simulink model "TEST_IPM_2_0"  (R2019b)
settings: configuration reference "Configuration" (kept outside this file)
PreLoadFcn:
  | RTWConfigurationCB('preloadfcn', bdroot);
values from neighbouring files (symbols this model uses):
  MParamFbase = 200.0    [TEST_IPM_LIB.sldd]
  MParamIbase = 360.0    [TEST_IPM_LIB.sldd]
  MParamLd = 0.002    [TEST_IPM_LIB.sldd]
  MParamLq = 0.002    [TEST_IPM_LIB.sldd]
  MParamRs = 1.15    [TEST_IPM_LIB.sldd]
  PWM_TPBRD_HALF = 5000.0    [TEST_IPM_LIB.sldd]
  Ts_10kHz = 0.0001    [TEST_IPM_LIB.sldd]
  Ts_1kHz = 0.001    [TEST_IPM_LIB.sldd]
undefined symbols (not defined in the file or in its folder): Down, GPTRIP1SEL, GPTRIP2SEL, TZ1, TZ2, Up
libraries: c280xlib x66, c2837xDlib x18, c2802xlib x10, powerlib_meascontrol x9, dsparch4 x4, c2000lib x1, c2806xlib x1, idelinklib_common x1
(part 2 of 6)

== system TEST_IPM_2_0/BackgroundTask ==
  function : TriggerPort  TriggerType=function-call  VariantControl=Variant
  CAN Calibration Protocol : c280xlib/CAN Calibration Protocol  CCP_STATION_ID=hex2dec('1')  module=eCAN_A  ccp_cro_id=hex2dec('6FA')  ccp_cro_message_type=Standard (11-bit identifier)  ccp_return_id=hex2dec('6FB')  ccp_return_message_type=Standard (11-bit identifier)  TOTAL_NUM_ODTS=8  cro_sample_time=-1
      settings: SourceProductName=Embedded Coder Support Package for Texas Instruments C2000 Processors  SourceProductBaseCode=TIC2000

== system TEST_IPM_2_0/BufferOut ==
  MATLAB Function : MATLAB Function  TreatAsAtomicUnit=on

== system TEST_IPM_2_0/CLATask ==
  function : TriggerPort  TriggerType=function-call  VariantControl=Variant
  Data Store Read : DataStoreRead  DataStoreName=SMO_RsRated
  Data Store Read1 : DataStoreRead  DataStoreName=SMO_Ual
  Data Store Read10 : DataStoreRead  DataStoreName=SMO_T
  Data Store Read11 : DataStoreRead  DataStoreName=SMO_SatPhi
  Data Store Read12 : DataStoreRead  DataStoreName=SMO_LdRated
  Data Store Read13 : DataStoreRead  DataStoreName=SMO_LqRated
  Data Store Read14 : DataStoreRead  DataStoreName=SMO_we
  Data Store Read2 : DataStoreRead  DataStoreName=SMO_Ube
  Data Store Read3 : DataStoreRead  DataStoreName=SMO_IbeEst
  Data Store Read31 : DataStoreRead  DataStoreName=SMO_FLAG
  Data Store Read4 : DataStoreRead  DataStoreName=SMO_IalEst
  Data Store Read5 : DataStoreRead  DataStoreName=SMO_Ial
  Data Store Read6 : DataStoreRead  DataStoreName=SMO_Ibe
  Data Store Read7 : DataStoreRead  DataStoreName=SMO_EalEst
  Data Store Read8 : DataStoreRead  DataStoreName=SMO_EbeEst
  Data Store Read9 : DataStoreRead  DataStoreName=SMO_K
  Data Store Write10 : DataStoreWrite  DataStoreName=SMO_IbeEstOut
  Data Store Write18 : DataStoreWrite  DataStoreName=SMO_IalEst
  Data Store Write19 : DataStoreWrite  DataStoreName=SMO_IbeEst
  Data Store Write20 : DataStoreWrite  DataStoreName=SMO_EalEst
  Data Store Write21 : DataStoreWrite  DataStoreName=SMO_EbeEstOut
  Data Store Write4 : DataStoreWrite  DataStoreName=SMO_EalEstOut
  Data Store Write5 : DataStoreWrite  DataStoreName=SMO_EbeEst
  Data Store Write9 : DataStoreWrite  DataStoreName=SMO_IalEstOut
  Function-Call Subsystem : Subsystem  TreatAsAtomicUnit=on
  Function-Call Subsystem1 : Subsystem  TreatAsAtomicUnit=on
  MATLAB Function5 : MATLAB Function  TreatAsAtomicUnit=on
  MATLAB Function8 : MATLAB Function  TreatAsAtomicUnit=on
  wires:
  Data Store Read31/1 -> MATLAB Function8/1(FLAG)
  MATLAB Function8/1(SMOClear()) -> Function-Call Subsystem/Trigger
  Data Store Read1/1 -> MATLAB Function5/1(Ual)
  Data Store Read2/1 -> MATLAB Function5/2(Ube)
  Data Store Read5/1 -> MATLAB Function5/3(Ial)
  Data Store Read6/1 -> MATLAB Function5/4(Ibe)
  Data Store Read4/1 -> MATLAB Function5/5(IalEst)
  Data Store Read3/1 -> MATLAB Function5/6(IbeEst)
  Data Store Read7/1 -> MATLAB Function5/7(EalEst)
  Data Store Read8/1 -> MATLAB Function5/8(EbeEst)
  Data Store Read9/1 -> MATLAB Function5/13(K)
  Data Store Read10/1 -> MATLAB Function5/14(eta)
  Data Store Read11/1 -> MATLAB Function5/15(SatPsi)
  Data Store Read/1 -> MATLAB Function5/11(RsRated)
  Data Store Read12/1 -> MATLAB Function5/9(LdRated)
  Data Store Read13/1 -> MATLAB Function5/10(LqRated)
  Data Store Read14/1 -> MATLAB Function5/12(we)
  MATLAB Function5/2(IbeEstOut) -> Data Store Write19/1, Data Store Write10/1
  MATLAB Function5/3(EalEstOut) -> Data Store Write4/1, Data Store Write20/1
  MATLAB Function5/4(EbeEstOut) -> Data Store Write21/1, Data Store Write5/1
  MATLAB Function5/1(IalEstOut) -> Data Store Write9/1, Data Store Write18/1
  MATLAB Function8/2(SMO_V()) -> Function-Call Subsystem1/Trigger

== system TEST_IPM_2_0/INT ==
  function : TriggerPort  TriggerType=function-call  VariantControl=Variant
  AD2S1210 Init : Subsystem  TreatAsAtomicUnit=on
  Chart : Stateflow chart  BlockKeywords=__PRM__SERIALIZED__DATA__:Stateflow Chart,Stateflow Diagram  TreatAsAtomicUnit=on
  Constant : Constant  Value=0  OutDataTypeStr=uint16  SampleTime=-1
  Current Bias Init : Subsystem  TreatAsAtomicUnit=on
  Current Sampling : Subsystem  TreatAsAtomicUnit=on
  Data Buffer : Subsystem  TreatAsAtomicUnit=on
  Data Store Write : DataStoreWrite  DataStoreName=ChartFlag
  Data Store Write1 : DataStoreWrite  DataStoreName=FLAG_5742
  Extra Observer : Subsystem  TreatAsAtomicUnit=on
  GPIO Down : Subsystem  TreatAsAtomicUnit=on
  GPIO UP : Subsystem  TreatAsAtomicUnit=on
  MAX5742 : Subsystem  TreatAsAtomicUnit=on
  Motor Control : Subsystem  TreatAsAtomicUnit=on
  Read Rotor Position : Subsystem  TreatAsAtomicUnit=on
  ePWM : Subsystem  TreatAsAtomicUnit=on
  wires:
  Constant/1 -> Data Store Write1/1, Data Store Write/1
  Chart/1(ADCINT_IN()) -> GPIO UP/Trigger
  Chart/2(ADCSample()) -> Current Sampling/Trigger
  Chart/5(AD2S1210()) -> Read Rotor Position/Trigger
  Chart/11(ADCINT_OUT()) -> GPIO Down/Trigger
  Chart/3(INIT_AD2S1210()) -> AD2S1210 Init/Trigger
  Chart/4(INIT_ADBias()) -> Current Bias Init/Trigger
  Chart/8(ePWM()) -> ePWM/Trigger
  Chart/6(MOTORCONTROL()) -> Motor Control/Trigger
  Chart/9(Buffer()) -> Data Buffer/Trigger
  Chart/10(DA_5742()) -> MAX5742/Trigger
  Chart/7(Extra_Observer()) -> Extra Observer/Trigger

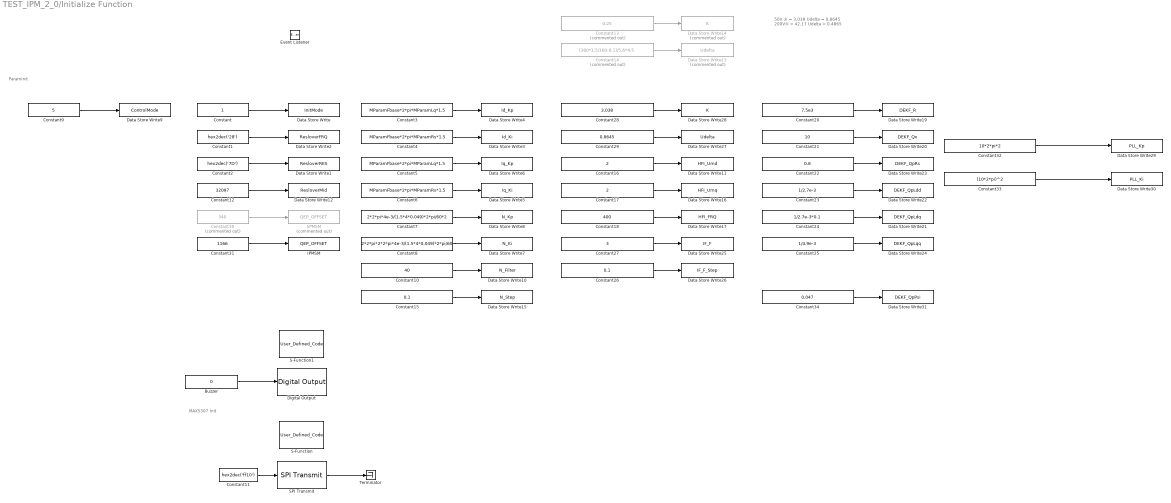
== system TEST_IPM_2_0/Initialize Function ==
  note: 50V  :k = 3.038 Udelta = 0.8645
      | 200V:k = 42.17 Udelta = 0.4865
  note: ParamInit
  note: MAX5307 Init
  Buzzer : Constant  Value=0  OutDataTypeStr=uint16  SampleTime=-1
  Constant : Constant  OutDataTypeStr=Inherit: Inherit via back propagation  SampleTime=-1
  Constant1 : Constant  Value=hex2dec('28')  OutDataTypeStr=Inherit: Inherit via back propagation  SampleTime=-1
  Constant10 : Constant  Value=40  OutDataTypeStr=Inherit: Inherit via back propagation  SampleTime=-1
  Constant11 : Constant  Priority=7  Value=hex2dec('ff10')  OutDataTypeStr=uint16  SampleTime=-1
  Constant12 : Constant  Value=32097  OutDataTypeStr=Inherit: Inherit via back propagation  SampleTime=-1
  Constant13 : Constant  Commented=on  Value=0.25  OutDataTypeStr=Inherit: Inherit via back propagation  SampleTime=-1
  Constant14 : Constant  Commented=on  Value=(380*1.5/100-0.1)/5.6*4.5  OutDataTypeStr=Inherit: Inherit via back propagation  SampleTime=-1
  Constant15 : Constant  Value=0.1  OutDataTypeStr=Inherit: Inherit via back propagation  SampleTime=-1
  Constant16 : Constant  Value=2  OutDataTypeStr=Inherit: Inherit via back propagation  SampleTime=-1
  Constant17 : Constant  Value=2  OutDataTypeStr=Inherit: Inherit via back propagation  SampleTime=-1
  Constant18 : Constant  Value=400  OutDataTypeStr=Inherit: Inherit via back propagation  SampleTime=-1
  Constant2 : Constant  Value=hex2dec('7D')  OutDataTypeStr=Inherit: Inherit via back propagation  SampleTime=-1
  Constant20 : Constant  Value=7.5e3  OutDataTypeStr=Inherit: Inherit via back propagation  SampleTime=-1
  Constant21 : Constant  Value=10  OutDataTypeStr=Inherit: Inherit via back propagation  SampleTime=-1
  Constant22 : Constant  Value=0.8  OutDataTypeStr=Inherit: Inherit via back propagation  SampleTime=-1
  Constant23 : Constant  Value=1/2.7e-3  OutDataTypeStr=Inherit: Inherit via back propagation  SampleTime=-1
  Constant24 : Constant  Value=1/2.7e-3*0.1  OutDataTypeStr=Inherit: Inherit via back propagation  SampleTime=-1
  Constant25 : Constant  Value=1/4.9e-3  OutDataTypeStr=Inherit: Inherit via back propagation  SampleTime=-1
  Constant26 : Constant  Value=0.1  OutDataTypeStr=Inherit: Inherit via back propagation  SampleTime=-1
  Constant27 : Constant  Value=3  OutDataTypeStr=Inherit: Inherit via back propagation  SampleTime=-1
  Constant28 : Constant  Value=3.038  OutDataTypeStr=Inherit: Inherit via back propagation  SampleTime=-1
  Constant29 : Constant  Value=0.8645  OutDataTypeStr=Inherit: Inherit via back propagation  SampleTime=-1
  Constant3 : Constant  Value=MParamFbase*2*pi*MParamLq*1.5  OutDataTypeStr=Inherit: Inherit via back propagation  SampleTime=-1
  Constant30 : Constant  Commented=on  Value=340  OutDataTypeStr=Inherit: Inherit via back propagation  SampleTime=-1
  Constant31 : Constant  Value=1166  OutDataTypeStr=Inherit: Inherit via back propagation  SampleTime=-1
  Constant32 : Constant  Value=10*2*pi*2  OutDataTypeStr=Inherit: Inherit via back propagation  SampleTime=-1
  Constant33 : Constant  Value=(10*2*pi)^2  OutDataTypeStr=Inherit: Inherit via back propagation  SampleTime=-1
  Constant34 : Constant  Value=0.047  OutDataTypeStr=Inherit: Inherit via back propagation  SampleTime=-1
  Constant4 : Constant  Value=MParamFbase*2*pi*MParamRs*1.5  OutDataTypeStr=Inherit: Inherit via back propagation  SampleTime=-1
  Constant5 : Constant  Value=MParamFbase*2*pi*MParamLq*1.5  OutDataTypeStr=Inherit: Inherit via back propagation  SampleTime=-1
  Constant6 : Constant  Value=MParamFbase*2*pi*MParamRs*1.5  OutDataTypeStr=Inherit: Inherit via back propagation  SampleTime=-1
  Constant7 : Constant  Value=2*2*pi*4e-3/(1.5*4*0.049)*2*pi/60*2  OutDataTypeStr=Inherit: Inherit via back propagation  SampleTime=-1
  Constant8 : Constant  Value=2*2*pi*2*2*pi*4e-3/(1.5*4*0.049)*2*pi/60  OutDataTypeStr=Inherit: Inherit via back propagation  SampleTime=-1
  Constant9 : Constant  Value=5  OutDataTypeStr=Inherit: Inherit via back propagation  SampleTime=-1
  Data Store Write : DataStoreWrite  DataStoreName=InitMode
  Data Store Write1 : DataStoreWrite  DataStoreName=ResloverRES
  Data Store Write10 : DataStoreWrite  DataStoreName=N_Filter
  Data Store Write11 : DataStoreWrite  DataStoreName=HFI_Umd
  Data Store Write12 : DataStoreWrite  DataStoreName=ResloverMid
  Data Store Write13 : DataStoreWrite  Commented=on  DataStoreName=Udelta
  Data Store Write14 : DataStoreWrite  Commented=on  DataStoreName=K
  Data Store Write15 : DataStoreWrite  DataStoreName=N_Step
  Data Store Write16 : DataStoreWrite  DataStoreName=HFI_Umq
  Data Store Write17 : DataStoreWrite  DataStoreName=HFI_FRQ
  Data Store Write19 : DataStoreWrite  DataStoreName=DEKF_R
  Data Store Write2 : DataStoreWrite  DataStoreName=ResloverFRQ
  Data Store Write20 : DataStoreWrite  DataStoreName=DEKF_Qx
  Data Store Write21 : DataStoreWrite  DataStoreName=DEKF_QpLdq
  Data Store Write22 : DataStoreWrite  DataStoreName=DEKF_QpLdd
  Data Store Write23 : DataStoreWrite  DataStoreName=DEKF_QpRs
  Data Store Write24 : DataStoreWrite  DataStoreName=DEKF_QpLqq
  Data Store Write25 : DataStoreWrite  DataStoreName=IF_F
  Data Store Write26 : DataStoreWrite  DataStoreName=IF_F_Step
  Data Store Write27 : DataStoreWrite  DataStoreName=Udelta
  Data Store Write28 : DataStoreWrite  DataStoreName=K
  Data Store Write29 : DataStoreWrite  DataStoreName=PLL_Kp
  Data Store Write3 : DataStoreWrite  DataStoreName=Id_Ki
  Data Store Write30 : DataStoreWrite  DataStoreName=PLL_Ki
  Data Store Write31 : DataStoreWrite  DataStoreName=DEKF_QpPsi
  Data Store Write4 : DataStoreWrite  DataStoreName=Id_Kp
  Data Store Write5 : DataStoreWrite  DataStoreName=Iq_Ki
  Data Store Write6 : DataStoreWrite  DataStoreName=Iq_Kp
  Data Store Write7 : DataStoreWrite  DataStoreName=N_Ki
  Data Store Write8 : DataStoreWrite  DataStoreName=N_Kp
  Data Store Write9 : DataStoreWrite  DataStoreName=ControlMode
  Digital Output : c2837xDlib/Digital Output  GPIO_Number=GPIO32~GPIO39  GPIO_Bit0=off  GPIO_BIT0_Toggle=off  GPIO_Bit1=off  GPIO_BIT1_Toggle=off  GPIO_Bit2=on  GPIO_BIT2_Toggle=off  GPIO_Bit3=off  GPIO_BIT3_Toggle=off  GPIO_Bit4=off  GPIO_BIT4_Toggle=off  GPIO_Bit5=off  GPIO_BIT5_Toggle=off  GPIO_Bit6=off  GPIO_BIT6_Toggle=off  GPIO_Bit7=off  GPIO_BIT7_Toggle=off
      settings: SourceProductName=Embedded Coder Support Package for Texas Instruments C2000 Processors  SourceProductBaseCode=TIC2000
  Event Listener : EventListener  DisableCoverage=on  EventName=reset
  IPMSM : DataStoreWrite  DataStoreName=QEP_OFFSET
  S-Function : S-Function  Priority=0  FunctionName=User_Defined_Code  Parameters=code  SFunctionDeploymentMode=off  EnableBusSupport=off  mask{code=DELAY_US(5000L);}
  S-Function1 : S-Function  Priority=100  FunctionName=User_Defined_Code  Parameters=code  SFunctionDeploymentMode=off  EnableBusSupport=off  mask{code=__asm(" MSETFLG RNDF32=1");}
  SPI Transmit : c280xlib/SPI Transmit  SPISelect=SPI_B  ClockPolarity=Rising_edge  ClockPhase=No_delay  SPIModule=uint32(0)  Mode=Master  BusSpeed=uint32(1000000)  FirstBitToTransfer=Most significant bit (MSB)  ClockMode=0  BlockFunction=Write  EnableRegisterAddress=on  RegisterAddress=0  OutputDataType=int8  OutputDataLength=1  BlockingMode=off  DataBits=16  UseCustomSSPin=Provided by the SPI peripheral  ActiveLowSSPin=Active low  Pin=0
      settings: SourceProductName=Embedded Coder Support Package for Texas Instruments C2000 Processors  SourceProductBaseCode=TIC2000
  SPMSM : DataStoreWrite  Commented=on  DataStoreName=QEP_OFFSET
  Terminator : Terminator
  wires:
  Constant/1 -> Data Store Write/1
  Constant1/1 -> Data Store Write2/1
  Constant2/1 -> Data Store Write1/1
  Constant4/1 -> Data Store Write3/1
  Constant3/1 -> Data Store Write4/1
  Constant5/1 -> Data Store Write6/1
  Constant6/1 -> Data Store Write5/1
  Constant8/1 -> Data Store Write7/1
  Constant7/1 -> Data Store Write8/1
  Constant9/1 -> Data Store Write9/1
  Constant10/1 -> Data Store Write10/1
  Buzzer/1 -> Digital Output/1
  Constant12/1 -> Data Store Write12/1
  Constant13/1 -> Data Store Write14/1
  Constant14/1 -> Data Store Write13/1
  Constant15/1 -> Data Store Write15/1
  Constant11/1 -> SPI Transmit/1
  SPI Transmit/1 -> Terminator/1
  Constant20/1 -> Data Store Write19/1
  Constant21/1 -> Data Store Write20/1
  Constant22/1 -> Data Store Write23/1
  Constant23/1 -> Data Store Write22/1
  Constant24/1 -> Data Store Write21/1
  Constant25/1 -> Data Store Write24/1
  Constant16/1 -> Data Store Write11/1
  Constant17/1 -> Data Store Write16/1
  Constant18/1 -> Data Store Write17/1
  Constant26/1 -> Data Store Write26/1
  Constant27/1 -> Data Store Write25/1
  Constant29/1 -> Data Store Write27/1
  Constant28/1 -> Data Store Write28/1
  Constant30/1 -> SPMSM/1
  Constant31/1 -> IPMSM/1
  Constant32/1 -> Data Store Write29/1
  Constant33/1 -> Data Store Write30/1
  Constant34/1 -> Data Store Write31/1

== system TEST_IPM_2_0/SpeedREF ==
  note: SMO Param
  Data Store Read : DataStoreRead  DataStoreName=N_Dem
  Data Store Read1 : DataStoreRead  DataStoreName=N_FBK
  Data Store Read2 : DataStoreRead  DataStoreName=N_Step
  Data Store Read21 : DataStoreRead  DataStoreName=SMO_ThetaV
  Data Store Read3 : DataStoreRead  DataStoreName=PLL_BdGain
  Data Store Write : DataStoreWrite  DataStoreName=N_REF
  Data Store Write1 : DataStoreWrite  DataStoreName=SMO_n
  Data Store Write2 : DataStoreWrite  DataStoreName=SMO_we
  Data Store Write29 : DataStoreWrite  DataStoreName=PLL_Kp
  Data Store Write30 : DataStoreWrite  DataStoreName=PLL_Ki
  Data Store Write6 : DataStoreWrite  DataStoreName=SMO_K
  Data Store Write7 : DataStoreWrite  DataStoreName=SMO_T
  "First Order Filter " : Subsystem
  Gain : Gain  Gain=2*pi*4/60  OutDataTypeStr=single
  Gain1 : Gain  Gain=5/60*2*pi
  Gain2 : Gain  Gain=2
  MATLAB Function1 : MATLAB Function  TreatAsAtomicUnit=on
  MATLAB Function3 : MATLAB Function  TreatAsAtomicUnit=on
  Product : Product
  Saturation : Saturate  UpperLimit=6000  LowerLimit=-6000
  Saturation1 : Saturate  UpperLimit=6000  LowerLimit=-6000
  Saturation2 : Saturate  UpperLimit=10*2*pi  LowerLimit=0.1*2*pi
  Square : Math  Operator=square  SignedPower=off  SaturateOnIntegerOverflow=on
  Subsystem1 : Subsystem
  Unit Delay : UnitDelay  SampleTime=-1  HasFrameUpgradeWarning=on
  wires:
  Data Store Read/1 -> Saturation/1
  Data Store Read2/1 -> Subsystem1/2(Step)
  Subsystem1/1(RampOutput) -> Saturation1/1
  Saturation/1 -> Subsystem1/1(TargetValue)
  Unit Delay/1 -> MATLAB Function1/2(theta_old)
  MATLAB Function1/1(speed) -> "First Order Filter "/1(input)
  Data Store Read21/1 -> MATLAB Function1/1(theta), Unit Delay/1
  "First Order Filter "/1("output ") -> Data Store Write1/1
  Data Store Read1/1 -> Gain/1
  Gain/1 -> Data Store Write2/1
  Saturation1/1 -> Gain1/1, MATLAB Function3/1(nREF), Data Store Write/1
  Gain1/1 -> Saturation2/1
  Product/1 -> Square/1, Gain2/1
  Gain2/1 -> Data Store Write29/1
  Square/1 -> Data Store Write30/1
  Saturation2/1 -> Product/1
  Data Store Read3/1 -> Product/2
  MATLAB Function3/1(K) -> Data Store Write6/1
  MATLAB Function3/2(T) -> Data Store Write7/1

== system TEST_IPM_2_0/Subsystem ==
  note: 更新了程序执行流程
      | 1.状态机设计程序执行时序
      | 2.中断内部状态机初始化AD2S1210，目前可以实现激励频率修改和故障码读取
      |    2.1分辨率需要修改硬件电阻，目前还未更改
      | 3.位置锁存在AD采样同时，防止系统延迟造成误差
      | 4.PWM硬件是反的，pwmA是下管，pwmB是上管，所以采用upcount时CLEAR,
      |    downcount时SET，然后pwmB反向

== system TEST_IPM_2_0/Temperature&DCBUS ==
  note: UdqFilter
  ADC_TempA : c2802xlib/ADC  blkParamProc=C2000_Type4  ADCModule=A  samplingMode=Single sample mode  ADCResolution=12-bit (Single-ended input)  useSOC1=SOC3  useSOC2=SOC0_SOC1  SOCAcquisitionWindow=15  SOCTriggerSource=Software  SOCInterruptTrigger=No ADCINT  Ts=0.02  dType=uint16  postInterrupt=off  interruptSel=ADCINT1  ADCINTContinuous=on  endma=off  chdma=1  conv1=ADCINA0  conv2=ADCINA0 and ADCINB0  conv1_Type4=ADCIN3  conv2_Type4=ADCIN0 and ADCIN1
      settings: SourceProductName=Embedded Coder Support Package for Texas Instruments C2000 Processors
  ADC_TempB : c2802xlib/ADC  blkParamProc=C2000_Type4  ADCModule=A  samplingMode=Single sample mode  ADCResolution=12-bit (Single-ended input)  useSOC1=SOC4  useSOC2=SOC0_SOC1  SOCAcquisitionWindow=15  SOCTriggerSource=Software  SOCInterruptTrigger=No ADCINT  Ts=0.02  dType=uint16  postInterrupt=off  interruptSel=ADCINT1  ADCINTContinuous=on  endma=off  chdma=1  conv1=ADCINA0  conv2=ADCINA0 and ADCINB0  conv1_Type4=ADCIN1  conv2_Type4=ADCIN0 and ADCIN1
      settings: SourceProductName=Embedded Coder Support Package for Texas Instruments C2000 Processors
  ADC_TempC : c2802xlib/ADC  blkParamProc=C2000_Type4  ADCModule=A  samplingMode=Single sample mode  ADCResolution=12-bit (Single-ended input)  useSOC1=SOC5  useSOC2=SOC0_SOC1  SOCAcquisitionWindow=15  SOCTriggerSource=Software  SOCInterruptTrigger=No ADCINT  Ts=0.02  dType=uint16  postInterrupt=off  interruptSel=ADCINT1  ADCINTContinuous=on  endma=off  chdma=1  conv1=ADCINA0  conv2=ADCINA0 and ADCINB0  conv1_Type4=ADCIN2  conv2_Type4=ADCIN0 and ADCIN1
      settings: SourceProductName=Embedded Coder Support Package for Texas Instruments C2000 Processors
  ADC_Udc : c2802xlib/ADC  blkParamProc=C2000_Type4  ADCModule=A  samplingMode=Single sample mode  ADCResolution=12-bit (Single-ended input)  useSOC1=SOC6  useSOC2=SOC0_SOC1  SOCAcquisitionWindow=15  SOCTriggerSource=Software  SOCInterruptTrigger=No ADCINT  Ts=0.001  dType=uint16  postInterrupt=off  interruptSel=ADCINT1  ADCINTContinuous=on  endma=off  chdma=1  conv1=ADCINA0  conv2=ADCINA0 and ADCINB0  conv1_Type4=ADCIN4  conv2_Type4=ADCIN0 and ADCIN1
      settings: SourceProductName=Embedded Coder Support Package for Texas Instruments C2000 Processors
  Data Store Read : DataStoreRead  DataStoreName=N_REF
  Data Store Read1 : DataStoreRead  DataStoreName=N_FBK
  Data Store Read2 : DataStoreRead  DataStoreName=ControlMode
  Data Store Read3 : DataStoreRead  DataStoreName=Id_REF
  Data Store Read4 : DataStoreRead  DataStoreName=UDOUT_Comp
  Data Store Read5 : DataStoreRead  DataStoreName=UQOUT_Comp
  Data Store Read6 : DataStoreRead  DataStoreName=USOUT_Comp
  Data Store Read7 : DataStoreRead  DataStoreName=Iq_REF
  Data Store Write : DataStoreWrite  DataStoreName=TempA
  Data Store Write1 : DataStoreWrite  DataStoreName=TempB
  Data Store Write2 : DataStoreWrite  DataStoreName=TempC
  Data Store Write3 : DataStoreWrite  DataStoreName=UDC
  Data Store Write4 : DataStoreWrite  DataStoreName=UdComP_Filter
  Data Store Write5 : DataStoreWrite  DataStoreName=UqComP_Filter
  Data Store Write6 : DataStoreWrite  DataStoreName=UsComP_Filter
  Data Store Write7 : DataStoreWrite  DataStoreName=Id_Filter
  Data Store Write8 : DataStoreWrite  DataStoreName=Iq_Filter
  First-Order Filter : powerlib_meascontrol/Filters/First-Order Filter  FilterType=Lowpass  Tc=1/10  Ts=0.02  Initialize=off  Vac_Init=[0, 0, 60]  Vdc_Init=0  PlotResponse=off  FreqRange="[0,  200,  1]"
      settings: SourceProductName=Simscape Electrical
  First-Order Filter1 : powerlib_meascontrol/Filters/First-Order Filter  FilterType=Lowpass  Tc=1/10  Ts=0.02  Initialize=off  Vac_Init=[0, 0, 60]  Vdc_Init=0  PlotResponse=off  FreqRange="[0,  200,  1]"
      settings: SourceProductName=Simscape Electrical
  First-Order Filter2 : powerlib_meascontrol/Filters/First-Order Filter  FilterType=Lowpass  Tc=1/10  Ts=0.02  Initialize=off  Vac_Init=[0, 0, 60]  Vdc_Init=0  PlotResponse=off  FreqRange="[0,  200,  1]"
      settings: SourceProductName=Simscape Electrical
  First-Order Filter3 : powerlib_meascontrol/Filters/First-Order Filter  FilterType=Lowpass  Tc=1e-2  Ts=1/1e3  Initialize=off  Vac_Init=[0, 0, 60]  Vdc_Init=0  PlotResponse=off  FreqRange="[0,  200,  1]"
      settings: SourceProductName=Simscape Electrical
  First-Order Filter{4..8} (5 alike) : powerlib_meascontrol/Filters/First-Order Filter  FilterType=Lowpass  Tc=5  Ts=0.02  Initialize=off  Vac_Init=[0, 0, 60]  Vdc_Init=0  PlotResponse=off  FreqRange="[0,  200,  1]"
      settings: SourceProductName=Simscape Electrical
  MATLAB Function : MATLAB Function  TreatAsAtomicUnit=on
  MATLAB Function1 : MATLAB Function  TreatAsAtomicUnit=on
  MATLAB Function2 : MATLAB Function  TreatAsAtomicUnit=on
  MATLAB Function3 : MATLAB Function  TreatAsAtomicUnit=on
  MATLAB Function4 : MATLAB Function  TreatAsAtomicUnit=on
  Max : MinMax  Function=max  Inputs=3
  wires:
  ADC_TempC/1 -> MATLAB Function4/1(input)
  ADC_TempB/1 -> MATLAB Function2/1(input)
  ADC_TempA/1 -> MATLAB Function1/1(input)
  ADC_Udc/1 -> MATLAB Function/1(input)
  MATLAB Function1/1(Output) -> First-Order Filter/1
  MATLAB Function2/1(Output) -> First-Order Filter1/1
  MATLAB Function4/1(Output) -> First-Order Filter2/1
  MATLAB Function/1(Output) -> First-Order Filter3/1
  First-Order Filter/1 -> Data Store Write/1, Max/1
  First-Order Filter1/1 -> Data Store Write1/1, Max/2
  Max/1 -> MATLAB Function3/1(Temp_Max)
  First-Order Filter2/1 -> Data Store Write2/1, Max/3
  First-Order Filter3/1 -> Data Store Write3/1, MATLAB Function3/2(UDC)
  Data Store Read/1 -> MATLAB Function3/3(N_REF)
  Data Store Read1/1 -> MATLAB Function3/4(N_FBK)
  Data Store Read4/1 -> First-Order Filter4/1
  First-Order Filter4/1 -> Data Store Write4/1
  Data Store Read5/1 -> First-Order Filter5/1
  First-Order Filter5/1 -> Data Store Write5/1
  Data Store Read6/1 -> First-Order Filter6/1
  First-Order Filter6/1 -> Data Store Write6/1
  Data Store Read2/1 -> MATLAB Function3/5(ControlMode)
  First-Order Filter8/1 -> Data Store Write8/1
  Data Store Read7/1 -> First-Order Filter8/1
  First-Order Filter7/1 -> Data Store Write7/1
  Data Store Read3/1 -> First-Order Filter7/1

== system TEST_IPM_2_0/CLATask/Function-Call Subsystem ==
  function : TriggerPort  TriggerType=function-call  VariantControl=Variant
  Data Store Read : DataStoreRead  DataStoreName=SMO_LdIn
  Data Store Read1 : DataStoreRead  DataStoreName=SMO_Ual
  Data Store Read2 : DataStoreRead  DataStoreName=SMO_Ube
  Data Store Read3 : DataStoreRead  DataStoreName=SMO_RsIn
  Data Store Read4 : DataStoreRead  DataStoreName=SMO_LqIn
  Data Store Read5 : DataStoreRead  DataStoreName=SMO_RsVIn
  Data Store Read6 : DataStoreRead  DataStoreName=SMO_LqIn
  Data Store Read7 : DataStoreRead  DataStoreName=SMO_Ial
  Data Store Read8 : DataStoreRead  DataStoreName=SMO_Ibe
  Data Store Write : DataStoreWrite  DataStoreName=SMO_EalEstOut
  Data Store Write1 : DataStoreWrite  DataStoreName=SMO_EbeEst
  Data Store Write10 : DataStoreWrite  DataStoreName=SMO_LqV
  Data Store Write2 : DataStoreWrite  DataStoreName=SMO_EalEst
  Data Store Write3 : DataStoreWrite  DataStoreName=SMO_IalEst
  Data Store Write4 : DataStoreWrite  DataStoreName=SMO_RsRated
  Data Store Write5 : DataStoreWrite  DataStoreName=SMO_LdRated
  Data Store Write6 : DataStoreWrite  DataStoreName=SMO_IbeEst
  Data Store Write7 : DataStoreWrite  DataStoreName=SMO_EbeEstOut
  Data Store Write8 : DataStoreWrite  DataStoreName=SMO_LqRated
  Data Store Write9 : DataStoreWrite  DataStoreName=SMO_RsV
  wires:
  Data Store Read3/1 -> Data Store Write4/1
  Data Store Read4/1 -> Data Store Write8/1
  Data Store Read/1 -> Data Store Write5/1
  Data Store Read5/1 -> Data Store Write9/1
  Data Store Read6/1 -> Data Store Write10/1
  Data Store Read7/1 -> Data Store Write3/1
  Data Store Read8/1 -> Data Store Write6/1
  Data Store Read1/1 -> Data Store Write/1, Data Store Write2/1
  Data Store Read2/1 -> Data Store Write7/1, Data Store Write1/1

== system TEST_IPM_2_0/CLATask/Function-Call Subsystem1 ==
  function : TriggerPort  TriggerType=function-call  VariantControl=Variant
  Data Store Read10 : DataStoreRead  DataStoreName=SMO_LqVIn
  Data Store Read9 : DataStoreRead  DataStoreName=SMO_RsVIn
  Data Store Write11 : DataStoreWrite  DataStoreName=SMO_RsRated
  Data Store Write12 : DataStoreWrite  DataStoreName=SMO_LqRated
  Data Store Write13 : DataStoreWrite  DataStoreName=SMO_RsV
  Data Store Write14 : DataStoreWrite  DataStoreName=SMO_LqV
  wires:
  Data Store Read9/1 -> Data Store Write13/1, Data Store Write11/1
  Data Store Read10/1 -> Data Store Write14/1, Data Store Write12/1

== system TEST_IPM_2_0/INT/AD2S1210 Init ==
  function : TriggerPort  TriggerType=function-call  VariantControl=Variant
  AD2S1210 : Stateflow chart  BlockKeywords=__PRM__SERIALIZED__DATA__:Stateflow Chart,Stateflow Diagram  TreatAsAtomicUnit=on
  Function-Call Subsystem : Subsystem  TreatAsAtomicUnit=on
  Function-Call Subsystem1 : Subsystem  TreatAsAtomicUnit=on
  Function-Call Subsystem2 : Subsystem  TreatAsAtomicUnit=on
  Function-Call Subsystem3 : Subsystem  TreatAsAtomicUnit=on
  Function-Call Subsystem4 : Subsystem  TreatAsAtomicUnit=on
  wires:
  AD2S1210/1(EV_RESET()) -> Function-Call Subsystem/Trigger
  AD2S1210/3(WRITE_SPI_STEP1()) -> Function-Call Subsystem1/Trigger
  AD2S1210/4(WRITE_SPI_STEP2()) -> Function-Call Subsystem2/Trigger
  AD2S1210/2(ConfigMode()) -> Function-Call Subsystem3/Trigger
  AD2S1210/5(INIT_FINISH()) -> Function-Call Subsystem4/Trigger

== system TEST_IPM_2_0/INT/Current Bias Init ==
  note: SMO Param Init
  function : TriggerPort  TriggerType=function-call  VariantControl=Variant
  Add1 : Sum  OutDataTypeStr=Inherit: Inherit via back propagation
  Add2 : Sum  OutDataTypeStr=Inherit: Inherit via back propagation
  Add6 : Sum  OutDataTypeStr=Inherit: Inherit via back propagation
  Constant15 : Constant  Value=2.7e-3  OutDataTypeStr=Inherit: Inherit via back propagation  SampleTime=-1
  Constant26 : Constant  Value=-800  OutDataTypeStr=Inherit: Inherit via back propagation  SampleTime=-1
  Constant27 : Constant  Value=-10  OutDataTypeStr=Inherit: Inherit via back propagation  SampleTime=-1
  Constant28 : Constant  Value=0.93  OutDataTypeStr=Inherit: Inherit via back propagation  SampleTime=-1
  Constant29 : Constant  Value=4.9e-3  OutDataTypeStr=Inherit: Inherit via back propagation  SampleTime=-1
  Constant5 : Constant  Value=0.01  OutDataTypeStr=Inherit: Inherit via back propagation  SampleTime=-1
  Data Store Read : DataStoreRead  DataStoreName=U_AD
  Data Store Read1 : DataStoreRead  DataStoreName=V_AD
  Data Store Read2 : DataStoreRead  DataStoreName=W_AD
  Data Store Write : DataStoreWrite  DataStoreName=U_OFFSET
  Data Store Write1 : DataStoreWrite  DataStoreName=V_OFFSET
  Data Store Write10 : DataStoreWrite  DataStoreName=SMO_SatPhi
  Data Store Write2 : DataStoreWrite  DataStoreName=W_OFFSET
  Data Store Write20 : DataStoreWrite  DataStoreName=SMO_LdIn
  Data Store Write25 : DataStoreWrite  DataStoreName=SMO_K
  Data Store Write26 : DataStoreWrite  DataStoreName=SMO_T
  Data Store Write3 : DataStoreWrite  DataStoreName=InitMode
  Data Store Write4 : DataStoreWrite  DataStoreName=SMO_RsIn
  Data Store Write5 : DataStoreWrite  DataStoreName=SMO_LqIn
  Data Store Write6 : DataStoreWrite  DataStoreName=SMO_RsVIn
  Data Store Write7 : DataStoreWrite  DataStoreName=SMO_LqVIn
  Gain : Gain  Gain=2*pi*Ts_10kHz  OutDataTypeStr=single
  Gain1 : Gain  Gain=2*pi*Ts_10kHz  OutDataTypeStr=single
  Gain2 : Gain  Gain=2*pi*Ts_10kHz  OutDataTypeStr=single
  Gain3 : Gain  Gain=1-2*pi*Ts_10kHz  OutDataTypeStr=single
  Gain4 : Gain  Gain=1-2*pi*Ts_10kHz  OutDataTypeStr=single
  Gain5 : Gain  Gain=1-2*pi*Ts_10kHz  OutDataTypeStr=single
  MATLAB Function : MATLAB Function  TreatAsAtomicUnit=on
  Unit Delay1 : UnitDelay  SampleTime=-1  HasFrameUpgradeWarning=on
  Unit Delay2 : UnitDelay  SampleTime=-1  HasFrameUpgradeWarning=on
  Unit Delay6 : UnitDelay  SampleTime=-1  HasFrameUpgradeWarning=on
  wires:
  Data Store Read/1 -> Gain/1
  Data Store Read1/1 -> Gain1/1
  Data Store Read2/1 -> Gain2/1
  Add6/1 -> Data Store Write/1, Gain3/1
  Unit Delay6/1 -> Add6/2
  Gain/1 -> Add6/1
  Gain3/1 -> Unit Delay6/1
  Gain4/1 -> Unit Delay1/1
  Gain1/1 -> Add1/1
  Unit Delay1/1 -> Add1/2
  Add1/1 -> Data Store Write1/1, Gain4/1
  Add2/1 -> Data Store Write2/1, Gain5/1
  Unit Delay2/1 -> Add2/2
  Gain5/1 -> Unit Delay2/1
  Gain2/1 -> Add2/1
  MATLAB Function/1(InitMode) -> Data Store Write3/1
  Constant26/1 -> Data Store Write26/1
  Constant29/1 -> Data Store Write7/1, Data Store Write5/1
  Constant27/1 -> Data Store Write25/1
  Constant28/1 -> Data Store Write6/1, Data Store Write4/1
  Constant5/1 -> Data Store Write10/1
  Constant15/1 -> Data Store Write20/1

== system TEST_IPM_2_0/INT/Current Sampling ==
  note: 1/4095*3*1e3/4*2/500*200/6
  note: needing Calibration
  function : TriggerPort  TriggerType=function-call  VariantControl=Variant
  ADC_Wind1_U : c2802xlib/ADC  Priority=3  blkParamProc=C2000_Type4  ADCModule=B  samplingMode=Single sample mode  ADCResolution=12-bit (Single-ended input)  useSOC1=SOC0  useSOC2=SOC0_SOC1  SOCAcquisitionWindow=7  SOCTriggerSource=ePWM1_ADCSOCA  SOCInterruptTrigger=No ADCINT  Ts=-1  dType=uint16  postInterrupt=off  interruptSel=ADCINT1  ADCINTContinuous=off  endma=off  chdma=1  conv1=ADCINA0  conv2=ADCINA0 and ADCINB0  conv1_Type4=ADCIN0  conv2_Type4=ADCIN0 and ADCIN1
      settings: SourceProductName=Embedded Coder Support Package for Texas Instruments C2000 Processors
  ADC_Wind1_V : c2802xlib/ADC  Priority=5  blkParamProc=C2000_Type4  ADCModule=B  samplingMode=Single sample mode  ADCResolution=12-bit (Single-ended input)  useSOC1=SOC1  useSOC2=SOC0_SOC1  SOCAcquisitionWindow=7  SOCTriggerSource=ePWM1_ADCSOCA  SOCInterruptTrigger=No ADCINT  Ts=-1  dType=uint16  postInterrupt=off  interruptSel=ADCINT1  ADCINTContinuous=off  endma=off  chdma=1  conv1=ADCINA0  conv2=ADCINA0 and ADCINB0  conv1_Type4=ADCIN1  conv2_Type4=ADCIN0 and ADCIN1
      settings: SourceProductName=Embedded Coder Support Package for Texas Instruments C2000 Processors
  ADC_Wind1_W : c2802xlib/ADC  Priority=7  blkParamProc=C2000_Type4  ADCModule=B  samplingMode=Single sample mode  ADCResolution=12-bit (Single-ended input)  useSOC1=SOC2  useSOC2=SOC0_SOC1  SOCAcquisitionWindow=7  SOCTriggerSource=ePWM1_ADCSOCA  SOCInterruptTrigger=No ADCINT  Ts=-1  dType=uint16  postInterrupt=on  interruptSel=ADCINT1  ADCINTContinuous=off  endma=off  chdma=1  conv1=ADCINA0  conv2=ADCINA0 and ADCINB0  conv1_Type4=ADCIN2  conv2_Type4=ADCIN0 and ADCIN1
      settings: SourceProductName=Embedded Coder Support Package for Texas Instruments C2000 Processors
  Add : Sum  Inputs=+-  AccumDataTypeStr=single
  Data Store Read2 : DataStoreRead  Priority=9  DataStoreName=U_OFFSET
  Data Store Read3 : DataStoreRead  DataStoreName=V_OFFSET
  Data Store Read4 : DataStoreRead  DataStoreName=W_OFFSET
  Data Store Write : DataStoreWrite  Priority=4  DataStoreName=U_AD
  Data Store Write1 : DataStoreWrite  DataStoreName=U_Current
  Data Store Write2 : DataStoreWrite  DataStoreName=V_Current
  Data Store Write3 : DataStoreWrite  DataStoreName=W_Current
  Data Store Write4 : DataStoreWrite  Priority=6  DataStoreName=V_AD
  Data Store Write5 : DataStoreWrite  Priority=8  DataStoreName=W_AD
  Demux : Demux  Outputs=3
  Digital Output1 : c2837xDlib/Digital Output  GPIO_Number=GPIO48~GPIO55  GPIO_Bit0=off  GPIO_BIT0_Toggle=off  GPIO_Bit1=off  GPIO_BIT1_Toggle=off  GPIO_Bit2=off  GPIO_BIT2_Toggle=off  GPIO_Bit3=off  GPIO_BIT3_Toggle=off  GPIO_Bit4=off  GPIO_BIT4_Toggle=off  GPIO_Bit5=off  GPIO_BIT5_Toggle=off  GPIO_Bit6=on  GPIO_BIT6_Toggle=off  GPIO_Bit7=off  GPIO_BIT7_Toggle=off
      settings: SourceProductName=Embedded Coder Support Package for Texas Instruments C2000 Processors  SourceProductBaseCode=TIC2000
  Digital Output2 : c2837xDlib/Digital Output  GPIO_Number=GPIO48~GPIO55  GPIO_Bit0=off  GPIO_BIT0_Toggle=off  GPIO_Bit1=off  GPIO_BIT1_Toggle=off  GPIO_Bit2=off  GPIO_BIT2_Toggle=off  GPIO_Bit3=off  GPIO_BIT3_Toggle=off  GPIO_Bit4=off  GPIO_BIT4_Toggle=off  GPIO_Bit5=on  GPIO_BIT5_Toggle=off  GPIO_Bit6=off  GPIO_BIT6_Toggle=off  GPIO_Bit7=off  GPIO_BIT7_Toggle=off
      settings: SourceProductName=Embedded Coder Support Package for Texas Instruments C2000 Processors  SourceProductBaseCode=TIC2000
  Gain : Gain  Gain=0.366300366300366*1.0057176*0.066666666666667  OutDataTypeStr=single
  MATLAB Function : MATLAB Function  TreatAsAtomicUnit=on
  Mux : Mux  Inputs=3
  Mux1 : Mux  Inputs=3
  ResloverSAMPLE : Constant  Priority=1  Value=0  OutDataTypeStr=Inherit: Inherit via back propagation  SampleTime=-1
  ResloverSAMPLE1 : Constant  Priority=6  Value=0  OutDataTypeStr=Inherit: Inherit via back propagation  SampleTime=-1
  wires:
  ADC_Wind1_W/1 -> Mux/3, Data Store Write5/1
  ADC_Wind1_U/1 -> Mux/1, Data Store Write/1
  ADC_Wind1_V/1 -> Mux/2, Data Store Write4/1
  ResloverSAMPLE/1 -> Digital Output1/1
  Mux/1 -> Add/1
  Mux1/1 -> Add/2
  Data Store Read2/1 -> Mux1/1
  Data Store Read3/1 -> Mux1/2
  Data Store Read4/1 -> Mux1/3
  Add/1 -> Gain/1
  Gain/1 -> Demux/1
  Demux/1 -> MATLAB Function/1(U), Data Store Write1/1
  Demux/2 -> MATLAB Function/2(V), Data Store Write2/1
  Demux/3 -> MATLAB Function/3(W), Data Store Write3/1
  ResloverSAMPLE1/1 -> Digital Output2/1

== system TEST_IPM_2_0/INT/Data Buffer ==
  function : TriggerPort  TriggerType=function-call  VariantControl=Variant
  Data Store Read : DataStoreRead  Commented=on  DataStoreName=UDOUT_Comp
  Data Store Read1 : DataStoreRead  Commented=on  DataStoreName=Iq_REF
  Data Store Read2 : DataStoreRead  Commented=on  DataStoreName=Id_REF
  Data Store Read3 : DataStoreRead  Commented=on  DataStoreName=UQOUT_Comp
  Data Store Read4 : DataStoreRead  Commented=on  DataStoreName=Id_FBK
  Data Store Read5 : DataStoreRead  Commented=on  DataStoreName=Iq_FBK
  Function-Call Split1 : FunctionCallSplit  NumOutputPorts=2
  Function-Call Split2 : FunctionCallSplit  NumOutputPorts=2
  Function-Call Subsystem : Subsystem  TreatAsAtomicUnit=on
  Function-Call Subsystem1 : Subsystem  TreatAsAtomicUnit=on
  MATLAB Function1 : MATLAB Function  TreatAsAtomicUnit=on
  Subsystem : Subsystem
  wires:
  MATLAB Function1/1(INTFunc()) -> Function-Call Split1/1
  Function-Call Split1/1 -> Subsystem/Trigger
  Function-Call Split1/2 -> Function-Call Split2/1
  Function-Call Split2/1 -> Function-Call Subsystem/Trigger
  Function-Call Split2/2 -> Function-Call Subsystem1/Trigger

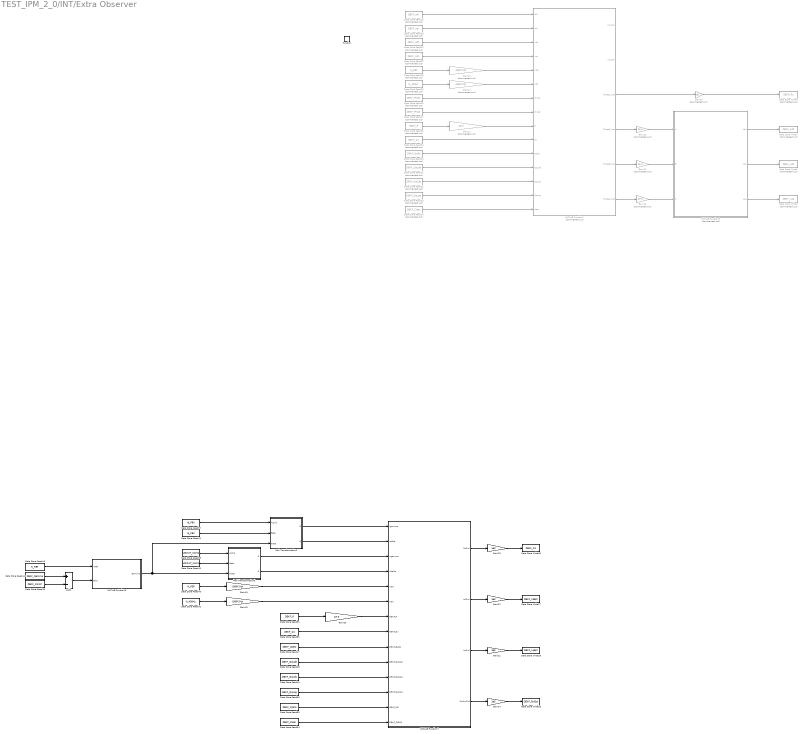
== system TEST_IPM_2_0/INT/Extra Observer ==
  function : TriggerPort  TriggerType=function-call  VariantControl=Variant  StatesWhenEnabling=reset
  Add1 : Sum  Inputs=+-
  Data Store Read19 : DataStoreRead  Commented=on  DataStoreName=DEKF_Idh
  Data Store Read20 : DataStoreRead  Commented=on  DataStoreName=DEKF_QpRs
  Data Store Read21 : DataStoreRead  Commented=on  DataStoreName=DEKF_QpLdd
  Data Store Read22 : DataStoreRead  Commented=on  DataStoreName=DEKF_QpLdq
  Data Store Read23 : DataStoreRead  Commented=on  DataStoreName=DEKF_QpLqq
  Data Store Read24 : DataStoreRead  Commented=on  DataStoreName=DEKF_Clear
  Data Store Read25 : DataStoreRead  Commented=on  DataStoreName=N_400Hz
  Data Store Read26 : DataStoreRead  Commented=on  DataStoreName=DEKF_Phid0
  Data Store Read27 : DataStoreRead  Commented=on  DataStoreName=DEKF_Phiq0
  Data Store Read29 : DataStoreRead  Commented=on  DataStoreName=N_REF
  Data Store Read30 : DataStoreRead  Commented=on  DataStoreName=DEKF_Iqh
  Data Store Read31 : DataStoreRead  Commented=on  DataStoreName=DEKF_Udh
  Data Store Read32 : DataStoreRead  Commented=on  DataStoreName=DEKF_Uqh
  Data Store Read33 : DataStoreRead  Commented=on  DataStoreName=DEKF_R
  Data Store Read34 : DataStoreRead  Commented=on  DataStoreName=DEKF_Qx
  Data Store Read37 : DataStoreRead  DataStoreName=Id_FBK
  Data Store Read39 : DataStoreRead  DataStoreName=UDOUT_Comp
  Data Store Read40 : DataStoreRead  DataStoreName=UQOUT_Comp
  Data Store Read41 : DataStoreRead  DataStoreName=Iq_FBK
  Data Store Read42 : DataStoreRead  DataStoreName=N_400Hz
  Data Store Read43 : DataStoreRead  DataStoreName=N_REF
  Data Store Read44 : DataStoreRead  DataStoreName=DEKF_Gamma
  Data Store Read45 : DataStoreRead  DataStoreName=DEKF_ComP
  Data Store Read46 : DataStoreRead  DataStoreName=N_REF
  Data Store Read47 : DataStoreRead  DataStoreName=DEKF_QpRs
  Data Store Read48 : DataStoreRead  DataStoreName=DEKF_QpLdd
  Data Store Read49 : DataStoreRead  DataStoreName=DEKF_QpLdq
  Data Store Read50 : DataStoreRead  DataStoreName=DEKF_QpLqq
  Data Store Read51 : DataStoreRead  DataStoreName=DEKF_R
  Data Store Read52 : DataStoreRead  DataStoreName=DEKF_Qx
  Data Store Read53 : DataStoreRead  DataStoreName=DEKF_QpPsi
  Data Store Read54 : DataStoreRead  DataStoreName=DEKF_Clear
  Data Store Write1 : DataStoreWrite  Commented=on  DataStoreName=DEKF_Ldd
  Data Store Write2 : DataStoreWrite  Commented=on  DataStoreName=DEKF_Ldq
  Data Store Write27 : DataStoreWrite  DataStoreName=DEKF_LdEst
  Data Store Write28 : DataStoreWrite  DataStoreName=DEKF_LqEst
  Data Store Write29 : DataStoreWrite  DataStoreName=DEKF_PsiEst
  Data Store Write3 : DataStoreWrite  Commented=on  DataStoreName=DEKF_Lqq
  Data Store Write30 : DataStoreWrite  DataStoreName=DEKF_Rs
  Data Store Write4 : DataStoreWrite  Commented=on  DataStoreName=DEKF_Rs
  Gain10 : Gain  Commented=on  Gain=4/60*2*pi
  Gain11 : Gain  Commented=on  Gain=1e-3
  Gain12 : Gain  Commented=on  Gain=4/60*2*pi
  Gain13 : Gain  Commented=on  Gain=1e-6
  Gain14 : Gain  Commented=on  Gain=1e-6
  Gain15 : Gain  Commented=on  Gain=1e-6
  Gain16 : Gain  Commented=on  Gain=1e3
  Gain18 : Gain  Gain=5/60*2*pi
  Gain19 : Gain  Gain=5/60*2*pi
  Gain20 : Gain  Gain=1e-3
  Gain{21..24} (4 alike) : Gain  Gain=1e3
  MATLAB Function1 : MATLAB Function  Commented=on  TreatAsAtomicUnit=on
  MATLAB Function3 : MATLAB Function  Commented=on  TreatAsAtomicUnit=on
  MATLAB Function7 : MATLAB Function  TreatAsAtomicUnit=on
  MATLAB Function8 : MATLAB Function  TreatAsAtomicUnit=on
  Park Transformation2 : Subsystem
  Park Transformation3 : Subsystem
  wires:
  Data Store Read22/1 -> MATLAB Function1/13(QpLdq)
  Gain12/1 -> MATLAB Function1/6(weh)
  Data Store Read33/1 -> Gain11/1
  Data Store Read34/1 -> MATLAB Function1/10(Qx)
  Gain11/1 -> MATLAB Function1/9(R)
  Data Store Read23/1 -> MATLAB Function1/14(QpLqq)
  Data Store Read25/1 -> Gain12/1
  Data Store Read30/1 -> MATLAB Function1/2(iqh)
  Data Store Read20/1 -> MATLAB Function1/11(QpRs)
  Data Store Read21/1 -> MATLAB Function1/12(QpLdd)
  Data Store Read24/1 -> MATLAB Function1/15(clear)
  Data Store Read31/1 -> MATLAB Function1/3(udh)
  Data Store Read29/1 -> Gain10/1
  Data Store Read27/1 -> MATLAB Function1/8(Phiq0)
  Data Store Read26/1 -> MATLAB Function1/7(Phid0)
  Data Store Read19/1 -> MATLAB Function1/1(idh)
  Data Store Read32/1 -> MATLAB Function1/4(uqh)
  Gain16/1 -> Data Store Write4/1
  Gain15/1 -> MATLAB Function3/3(C)
  Gain14/1 -> MATLAB Function3/2(B)
  Gain13/1 -> MATLAB Function3/1(A)
  MATLAB Function1/3(Theta1_hat) -> Gain16/1
  MATLAB Function3/3(Lqq) -> Data Store Write3/1
  MATLAB Function3/2(Ldq) -> Data Store Write2/1
  MATLAB Function3/1(Ldd) -> Data Store Write1/1
  MATLAB Function1/4(Theta2_hat) -> Gain13/1
  MATLAB Function1/5(Theta3_hat) -> Gain14/1
  MATLAB Function1/6(Theta4_hat) -> Gain15/1
  Gain10/1 -> MATLAB Function1/5(we0)
  Park Transformation2/1(D) -> MATLAB Function7/1(igamma)
  Park Transformation2/2(Q) -> MATLAB Function7/2(idelta)
  Park Transformation3/1(D) -> MATLAB Function7/3(ugamma)
  Park Transformation3/2(Q) -> MATLAB Function7/4(udelta)
  Data Store Read43/1 -> Gain18/1
  Data Store Read42/1 -> Gain19/1
  Gain18/1 -> MATLAB Function7/5(we0)
  Gain19/1 -> MATLAB Function7/6(weh)
  Data Store Read45/1 -> Add1/2
  MATLAB Function8/1(Gamma) -> Park Transformation3/3(theta), Park Transformation2/3(theta)
  Data Store Read44/1 -> Add1/1
  Add1/1 -> MATLAB Function8/2(Bias)
  Data Store Read46/1 -> MATLAB Function8/1(nRef)
  Data Store Read37/1 -> Park Transformation2/1(Alpha)
  Data Store Read41/1 -> Park Transformation2/2(Beta)
  Data Store Read39/1 -> Park Transformation3/1(Alpha)
  Data Store Read40/1 -> Park Transformation3/2(Beta)
  Data Store Read50/1 -> MATLAB Function7/12(DEKF_QpNqq)
  Data Store Read49/1 -> MATLAB Function7/11(DEKF_QpNdq)
  Data Store Read51/1 -> Gain20/1
  Data Store Read47/1 -> MATLAB Function7/9(DEKF_QpRs)
  Data Store Read48/1 -> MATLAB Function7/10(DEKF_QpNdd)
  Data Store Read52/1 -> MATLAB Function7/8(DEKF_Qx)
  Gain20/1 -> MATLAB Function7/7(DEKF_R)
  Data Store Read53/1 -> MATLAB Function7/13(DEKF_PSI)
  Data Store Read54/1 -> MATLAB Function7/14(DEKF_CLEAR)
  MATLAB Function7/1(RsOut) -> Gain23/1
  MATLAB Function7/2(LdOut) -> Gain22/1
  MATLAB Function7/3(LqOut) -> Gain21/1
  MATLAB Function7/4(PsidmOut) -> Gain24/1
  Gain21/1 -> Data Store Write28/1
  Gain22/1 -> Data Store Write27/1
  Gain23/1 -> Data Store Write30/1
  Gain24/1 -> Data Store Write29/1

== system TEST_IPM_2_0/INT/GPIO Down ==
  function : TriggerPort  TriggerType=function-call  VariantControl=Variant
  Constant : Constant  OutDataTypeStr=uint16  SampleTime=-1
  Digital Output : c2837xDlib/Digital Output  GPIO_Number=GPIO112~GPIO119  GPIO_Bit0=off  GPIO_BIT0_Toggle=off  GPIO_Bit1=on  GPIO_BIT1_Toggle=off  GPIO_Bit2=off  GPIO_BIT2_Toggle=off  GPIO_Bit3=off  GPIO_BIT3_Toggle=off  GPIO_Bit4=off  GPIO_BIT4_Toggle=off  GPIO_Bit5=off  GPIO_BIT5_Toggle=off  GPIO_Bit6=off  GPIO_BIT6_Toggle=off  GPIO_Bit7=off  GPIO_BIT7_Toggle=off
      settings: SourceProductName=Embedded Coder Support Package for Texas Instruments C2000 Processors  SourceProductBaseCode=TIC2000
  wires:
  Constant/1 -> Digital Output/1

== system TEST_IPM_2_0/INT/GPIO UP ==
  function : TriggerPort  TriggerType=function-call  VariantControl=Variant
  Add : Sum  Inputs=++++++
  Constant : Constant  Value=0  OutDataTypeStr=uint16  SampleTime=-1
  Data Store Write6 : DataStoreWrite  DataStoreName=IGBT_Fault
  Demux : Demux  Outputs=6
  Digital Input : c2837xDlib/Digital Input  GPIO_Number=GPIO40~GPIO47  GPIO_Bit0=on  GPIO_Bit1=on  GPIO_Bit2=off  GPIO_Bit3=off  GPIO_Bit4=on  GPIO_Bit5=on  GPIO_Bit6=on  GPIO_Bit7=on  sampleTime=-1  dataType=uint16  GPIO_Bit0_Qualification=Sync to SYSCLKOUT  GPIO_Bit1_Qualification=Sync to SYSCLKOUT  GPIO_Bit2_Qualification=Sync to SYSCLKOUT  GPIO_Bit3_Qualification=Sync to SYSCLKOUT  GPIO_Bit4_Qualification=Sync to SYSCLKOUT  GPIO_Bit5_Qualification=Sync to SYSCLKOUT  GPIO_Bit6_Qualification=Sync to SYSCLKOUT  GPIO_Bit7_Qualification=Sync to SYSCLKOUT  Qualification_Period=-1
      settings: SourceProductName=Embedded Coder Support Package for Texas Instruments C2000 Processors  SourceProductBaseCode=TIC2000
  Digital Output : c2837xDlib/Digital Output  GPIO_Number=GPIO112~GPIO119  GPIO_Bit0=off  GPIO_BIT0_Toggle=off  GPIO_Bit1=on  GPIO_BIT1_Toggle=off  GPIO_Bit2=off  GPIO_BIT2_Toggle=off  GPIO_Bit3=off  GPIO_BIT3_Toggle=off  GPIO_Bit4=off  GPIO_BIT4_Toggle=off  GPIO_Bit5=off  GPIO_BIT5_Toggle=off  GPIO_Bit6=off  GPIO_BIT6_Toggle=off  GPIO_Bit7=off  GPIO_BIT7_Toggle=off
      settings: SourceProductName=Embedded Coder Support Package for Texas Instruments C2000 Processors  SourceProductBaseCode=TIC2000
  Gain1 : Gain  Gain=2  OutDataTypeStr=uint16
  Gain2 : Gain  Gain=4  OutDataTypeStr=uint16
  Gain3 : Gain  Gain=8  OutDataTypeStr=uint16
  Gain4 : Gain  Gain=16  OutDataTypeStr=uint16
  Gain5 : Gain  Gain=32  OutDataTypeStr=uint16
  MATLAB Function2 : MATLAB Function  TreatAsAtomicUnit=on
  wires:
  Constant/1 -> Digital Output/1
  Gain4/1 -> Add/5
  Demux/1 -> Add/1
  Gain2/1 -> Add/3
  Demux/3 -> Gain2/1
  Demux/6 -> Gain5/1
  Demux/2 -> Gain1/1
  Demux/4 -> Gain3/1
  Demux/5 -> Gain4/1
  Gain5/1 -> Add/6
  Gain1/1 -> Add/2
  Gain3/1 -> Add/4
  Add/1 -> MATLAB Function2/1(IGBT_FAULT), Data Store Write6/1
  Digital Input/1 -> Demux/1
